simulink model "completed_model"  (R2026a)
settings: Solver=FixedStepDiscrete  StopTime=inf  FixedStep=0.01  EnableMultiTasking=on
undefined symbols (not defined in the file): dspblkCoreblockFVToolHelper, gcbh
libraries: arduinolib x7
settings Model: SILPILModeSetting=veronly  ExtModeTrigDuration=2  Creator=AdePratamaSuryoKusum  LastModifiedBy=AdePratamaSuryoKusum
settings DataIOCC: ExternalInput=milInput
settings HardwareCC: ProdBitPerInt=16.0  ProdBitPerPointer=16.0  ProdBitPerSizeT=16.0  ProdBitPerPtrDiffT=16.0  ProdWordSize=8.0  ProdHWDeviceType=Atmel->AVR
settings RTWCC: SystemTargetFile=ert.tlc  HardwareBoard=Arduino Uno  TLCOptions="-aInlineSetEventsForThisBaseRateFcn=TLC_FALSE -aSuppressMultiTaskScheduler=TLC_FALSE   -aRateBasedStepFcn=1"  Toolchain=Arduino AVR  BuildConfiguration=Faster Runs  Description=Embedded Coder
settings ERTTargetCC: ExtModeTransport=3.0  ExtModeAutomaticAllocSize=off  ExtModeStaticAllocSize=250.0  SupportContinuousTime=on  SupportVariableSizeSignals=on

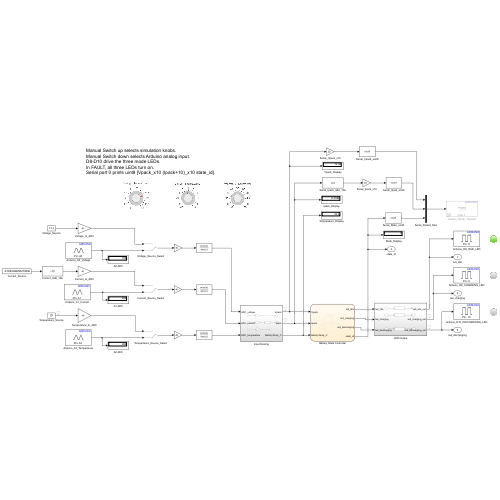
[thumbnail: Simulink's stored preview of the top-level diagram]
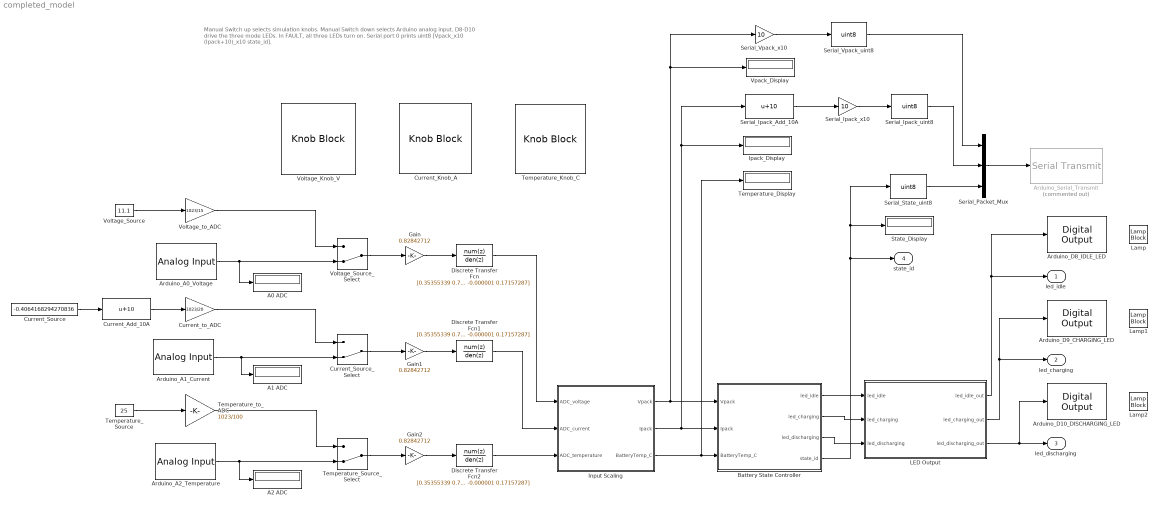
== system completed_model ==
  note: Manual Switch up selects simulation knobs.
      | Manual Switch down selects Arduino analog input.
      | D8-D10 drive the three mode LEDs.
      | In FAULT, all three LEDs turn on.
      | Serial port 0 prints uint8 [Vpack_x10 (Ipack+10)_x10 state_id].
  A0 ADC : Display
  A1 ADC : Display
  A2 ADC : Display
  Arduino_A0_Voltage : arduinolib/Analog Input  pinNumber=0  ReadResultsOnly=off  ConversionTriggerSource=Software  ExternalTriggerType=uint32( 0 )  OutputDataType=uint16  EnableConversionCompleteNotify=off  EnableOuputStatus=off  SampleTime=0.1  blockPlatform=arduino
  Arduino_A1_Current : arduinolib/Analog Input  pinNumber=1  ReadResultsOnly=off  ConversionTriggerSource=Software  ExternalTriggerType=uint32( 0 )  OutputDataType=uint16  EnableConversionCompleteNotify=off  EnableOuputStatus=off  SampleTime=0.1  blockPlatform=arduino
  Arduino_A2_Temperature : arduinolib/Analog Input  pinNumber=2  ReadResultsOnly=off  ConversionTriggerSource=Software  ExternalTriggerType=uint32( 0 )  OutputDataType=uint16  EnableConversionCompleteNotify=off  EnableOuputStatus=off  SampleTime=0.1  blockPlatform=arduino
  Arduino_D10_DISCHARGING_LED : arduinolib/Digital Output  pinNumber=10  Direction=output  blockPlatform=arduino
  Arduino_D8_IDLE_LED : arduinolib/Digital Output  pinNumber=8  Direction=output  blockPlatform=arduino
  Arduino_D9_CHARGING_LED : arduinolib/Digital Output  pinNumber=9  Direction=output  blockPlatform=arduino
  Arduino_Serial_Transmit : arduinolib/Serial Transmit  Commented=on  portNumber=0  sendmode=println  sendformat=Decimal  floatprecision=2  header=[]  terminator=[]  blockPlatform=ARDUINO
  Battery State Controller : Stateflow chart  TreatAsAtomicUnit=on
  Current_Add_10A : Bias  Bias=10  SaturateOnIntegerOverflow=off
  Current_Knob_A : KnobBlock  ScaleMin=-10  ScaleMax=10
  Current_Source : Constant  Value=-0.4064168294270836
  Current_Source_Select : ManualSwitch  CurrentSetting=0
  Current_to_ADC : Gain  Gain=1023/20
  Discrete Transfer Fcn : DiscreteTransferFcn  LoadFcn=dspblkCoreblockFVToolHelper(gcbh,'load');  Numerator=[0.35355339 0.70710678 0.35355339]  Denominator=[1 -0.000001 0.17157287]
      settings: CopyFcn=dspblkCoreblockFVToolHelper(gcbh,'copy');  DeleteFcn=dspblkCoreblockFVToolHelper(gcbh,'close');  ModelCloseFcn=dspblkCoreblockFVToolHelper(gcbh,'close');  PreSaveFcn=dspblkCoreblockFVToolHelper(gcbh,'presave');  PostSaveFcn=dspblkCoreblockFVToolHelper(gcbh,'postsave');  CloseFcn=dspblkCoreblockFVToolHelper(gcbh,'close');
  Discrete Transfer Fcn1 : DiscreteTransferFcn  LoadFcn=dspblkCoreblockFVToolHelper(gcbh,'load');  Numerator=[0.35355339 0.70710678 0.35355339]  Denominator=[1 -0.000001 0.17157287]
      settings: CopyFcn=dspblkCoreblockFVToolHelper(gcbh,'copy');  DeleteFcn=dspblkCoreblockFVToolHelper(gcbh,'close');  ModelCloseFcn=dspblkCoreblockFVToolHelper(gcbh,'close');  PreSaveFcn=dspblkCoreblockFVToolHelper(gcbh,'presave');  PostSaveFcn=dspblkCoreblockFVToolHelper(gcbh,'postsave');  CloseFcn=dspblkCoreblockFVToolHelper(gcbh,'close');
  Discrete Transfer Fcn2 : DiscreteTransferFcn  LoadFcn=dspblkCoreblockFVToolHelper(gcbh,'load');  Numerator=[0.35355339 0.70710678 0.35355339]  Denominator=[1 -0.000001 0.17157287]
      settings: CopyFcn=dspblkCoreblockFVToolHelper(gcbh,'copy');  DeleteFcn=dspblkCoreblockFVToolHelper(gcbh,'close');  ModelCloseFcn=dspblkCoreblockFVToolHelper(gcbh,'close');  PreSaveFcn=dspblkCoreblockFVToolHelper(gcbh,'presave');  PostSaveFcn=dspblkCoreblockFVToolHelper(gcbh,'postsave');  CloseFcn=dspblkCoreblockFVToolHelper(gcbh,'close');
  Gain : Gain  Gain=0.82842712
  Gain1 : Gain  Gain=0.82842712
  Gain2 : Gain  Gain=0.82842712
  Input Scaling : Subsystem
  Ipack_Display : Display
  LED Output : Subsystem
  Lamp : LampBlock  LabelPosition=Hide  DefaultColor=[192.0, 192.0, 192.0]
  Lamp1 : LampBlock  LabelPosition=Hide  DefaultColor=[192.0, 192.0, 192.0]
  Lamp2 : LampBlock  LabelPosition=Hide  DefaultColor=[192.0, 192.0, 192.0]
  Serial_Ipack_Add_10A : Bias  Bias=10  SaturateOnIntegerOverflow=off
  Serial_Ipack_uint8 : DataTypeConversion  OutDataTypeStr=uint8  SaturateOnIntegerOverflow=off  RndMeth=Floor
  Serial_Ipack_x10 : Gain  Gain=10
  Serial_Packet_Mux : Mux  Inputs=3
  Serial_State_uint8 : DataTypeConversion  OutDataTypeStr=uint8  SaturateOnIntegerOverflow=off  RndMeth=Floor
  Serial_Vpack_uint8 : DataTypeConversion  OutDataTypeStr=uint8  SaturateOnIntegerOverflow=off  RndMeth=Floor
  Serial_Vpack_x10 : Gain  Gain=10
  State_Display : Display
  Temperature_Display : Display
  Temperature_Knob_C : KnobBlock
  Temperature_Source : Constant  Value=25
  Temperature_Source_Select : ManualSwitch  CurrentSetting=0
  Temperature_to_ADC : Gain  Gain=1023/100
  Voltage_Knob_V : KnobBlock  ScaleMax=15
  Voltage_Source : Constant  Value=11.1
  Voltage_Source_Select : ManualSwitch  CurrentSetting=0
  Voltage_to_ADC : Gain  Gain=1023/15
  Vpack_Display : Display
  led_idle : Outport
  led_charging : Outport  Port=2
  led_discharging : Outport  Port=3
  state_id : Outport  Port=4
  wires:
  Current_Add_10A/1 -> Current_to_ADC/1
  Current_Source/1 -> Current_Add_10A/1
  Input Scaling/1(Vpack) -> Battery State Controller/1(Vpack), Serial_Vpack_x10/1, Vpack_Display/1
  Voltage_to_ADC/1 -> Voltage_Source_Select/1
  Voltage_Source_Select/1 -> Gain/1
  Voltage_Source/1 -> Voltage_to_ADC/1
  Temperature_Source_Select/1 -> Gain2/1
  Temperature_Source/1 -> Temperature_to_ADC/1
  Current_to_ADC/1 -> Current_Source_Select/1
  Temperature_to_ADC/1 -> Temperature_Source_Select/1
  Current_Source_Select/1 -> Gain1/1
  Input Scaling/2(Ipack) -> Ipack_Display/1, Serial_Ipack_Add_10A/1, Battery State Controller/2(Ipack)
  Input Scaling/3(BatteryTemp_C) -> Temperature_Display/1, Battery State Controller/3(BatteryTemp_C)
  Serial_Vpack_x10/1 -> Serial_Vpack_uint8/1
  Serial_Ipack_Add_10A/1 -> Serial_Ipack_x10/1
  Battery State Controller/1(led_idle) -> LED Output/1(led_idle)
  LED Output/2(led_charging_out) -> Arduino_D9_CHARGING_LED/1, led_charging/1
  Battery State Controller/2(led_charging) -> LED Output/2(led_charging)
  Battery State Controller/3(led_discharging) -> LED Output/3(led_discharging)
  Battery State Controller/4(state_id) -> Serial_State_uint8/1, State_Display/1, state_id/1
  Serial_Vpack_uint8/1 -> Serial_Packet_Mux/1
  Serial_State_uint8/1 -> Serial_Packet_Mux/3
  Serial_Ipack_x10/1 -> Serial_Ipack_uint8/1
  LED Output/1(led_idle_out) -> Arduino_D8_IDLE_LED/1, led_idle/1
  LED Output/3(led_discharging_out) -> led_discharging/1, Arduino_D10_DISCHARGING_LED/1
  Serial_Ipack_uint8/1 -> Serial_Packet_Mux/2
  Serial_Packet_Mux/1 -> Arduino_Serial_Transmit/1
  Arduino_A0_Voltage/1 -> A0 ADC/1, Voltage_Source_Select/2
  Arduino_A1_Current/1 -> A1 ADC/1, Current_Source_Select/2
  Arduino_A2_Temperature/1 -> A2 ADC/1, Temperature_Source_Select/2
  Discrete Transfer Fcn/1 -> Input Scaling/1(ADC_voltage)
  Discrete Transfer Fcn1/1 -> Input Scaling/2(ADC_current)
  Discrete Transfer Fcn2/1 -> Input Scaling/3(ADC_temperature)
  Gain/1 -> Discrete Transfer Fcn/1
  Gain1/1 -> Discrete Transfer Fcn1/1
  Gain2/1 -> Discrete Transfer Fcn2/1

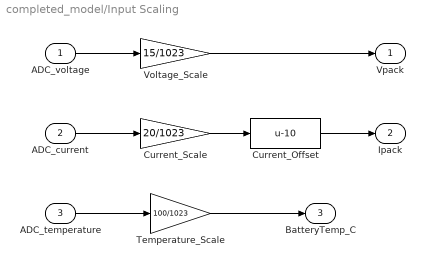
== system completed_model/Input Scaling ==
  ADC_voltage : Inport
  ADC_current : Inport  Port=2
  ADC_temperature : Inport  Port=3
  Current_Offset : Bias  Bias=-10  SaturateOnIntegerOverflow=off
  Current_Scale : Gain  Gain=20/1023
  Temperature_Scale : Gain  Gain=100/1023
  Voltage_Scale : Gain  Gain=15/1023
  Vpack : Outport
  Ipack : Outport  Port=2
  BatteryTemp_C : Outport  Port=3
  wires:
  ADC_voltage/1 -> Voltage_Scale/1
  Voltage_Scale/1 -> Vpack/1
  ADC_current/1 -> Current_Scale/1
  Current_Scale/1 -> Current_Offset/1
  Current_Offset/1 -> Ipack/1
  ADC_temperature/1 -> Temperature_Scale/1
  Temperature_Scale/1 -> BatteryTemp_C/1

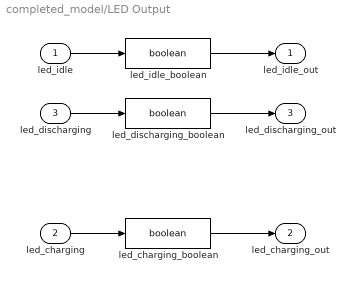
== system completed_model/LED Output ==
  led_idle : Inport
  led_charging : Inport  Port=2
  led_discharging : Inport  Port=3
  led_charging_boolean : DataTypeConversion  OutDataTypeStr=boolean  SaturateOnIntegerOverflow=off  RndMeth=Floor
  led_discharging_boolean : DataTypeConversion  OutDataTypeStr=boolean  SaturateOnIntegerOverflow=off  RndMeth=Floor
  led_idle_boolean : DataTypeConversion  OutDataTypeStr=boolean  SaturateOnIntegerOverflow=off  RndMeth=Floor
  led_idle_out : Outport
  led_charging_out : Outport  Port=2
  led_discharging_out : Outport  Port=3
  wires:
  led_charging/1 -> led_charging_boolean/1
  led_discharging/1 -> led_discharging_boolean/1
  led_idle/1 -> led_idle_boolean/1
  led_idle_boolean/1 -> led_idle_out/1
  led_discharging_boolean/1 -> led_discharging_out/1
  led_charging_boolean/1 -> led_charging_out/1

== stateflow chart completed_model/Battery State Controller ==
  state CHARGING
    during:
    led_idle=false; led_charging=true; led_discharging=false; state_id=uint8(1);
  state IDLE
    during:
    led_idle=true; led_charging=false; led_discharging=false; state_id=uint8(0);
  state FAULT
    during:
    led_idle=true; led_charging=true; led_discharging=true; state_id=uint8(3);
  state DISCHARGING
    during:
    led_idle=false; led_charging=false; led_discharging=true; state_id=uint8(2);
  DISCHARGING -> CHARGING [order 3] : [Ipack > 1.0 && Vpack >= 9.0 && Vpack <= 12.6]
  CHARGING -> FAULT [order 1] : [Vpack < 9.0 || Vpack > 12.6 || BatteryTemp_C > 50]
  CHARGING -> DISCHARGING [order 3] : [Ipack < -1.0 && Vpack >= 9.0 && Vpack <= 12.6]
  IDLE -> CHARGING [order 2] : [Ipack > 1.0 && Vpack >= 9.0 && Vpack <= 12.6]
  CHARGING -> IDLE [order 2] : [Ipack <= 1.0 && Ipack >= -1.0]
  (default) -> IDLE
  FAULT -> IDLE : [Vpack >= 9.0 && Vpack <= 12.6 && BatteryTemp_C <= 50 && Ipack >= -1.0 && Ipack <= 1.0]
  IDLE -> DISCHARGING [order 3] : [Ipack < -1.0 && Vpack >= 9.0 && Vpack <= 12.6]
  DISCHARGING -> IDLE [order 2] : [Ipack <= 1.0 && Ipack >= -1.0]
  IDLE -> FAULT [order 1] : [Vpack < 9.0 || Vpack > 12.6 || BatteryTemp_C > 50]
  DISCHARGING -> FAULT [order 1] : [Vpack < 9.0 || Vpack > 12.6 || BatteryTemp_C > 50]
  data: Vpack input double; Ipack input double; led_idle output boolean; led_charging output boolean; led_discharging output boolean; state_id output uint8; BatteryTemp_C input double
